simulink library "LibraryBlock"  (R2017b)
settings: Solver=VariableStepAuto  StartTime=0.0  StopTime=10.0  RelTol=1e-3
settings Model: Creator=minh  LastModifiedBy=minh

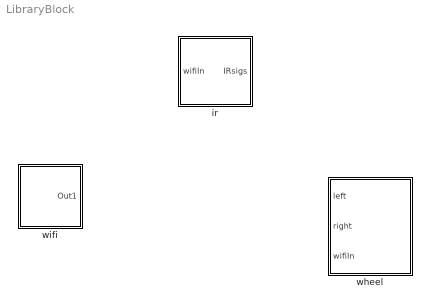
== system LibraryBlock ==
  "ir " : Subsystem
  wheel : Subsystem
  wifi : Subsystem

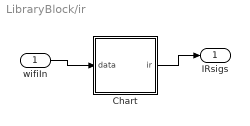
== system LibraryBlock/ir  ==
  wifiIn : Inport
  Chart : Stateflow chart  TreatAsAtomicUnit=on
  IRsigs : Outport
  wires:
  wifiIn/1 -> Chart/1(data)
  Chart/1(ir) -> IRsigs/1

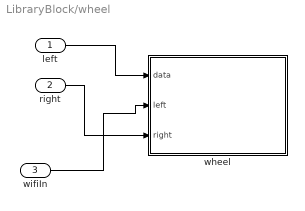
== system LibraryBlock/wheel ==
  left : Inport
  right : Inport  Port=2
  wifiIn : Inport  Port=3
  wheel : Stateflow chart  TreatAsAtomicUnit=on
  wires:
  left/1 -> wheel/1(data)
  right/1 -> wheel/3(right)
  wifiIn/1 -> wheel/2(left)

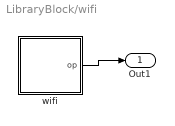
== system LibraryBlock/wifi ==
  wifi : Stateflow chart  TreatAsAtomicUnit=on
  Out1 : Outport
  wires:
  wifi/1(op) -> Out1/1

== stateflow chart LibraryBlock/wheel/wheel ==
  state f
    entry,during:
    wheel(right,left)
  (default) -> f
  data: u1 function_input; u2 function_input; data input; left input; right input
  function wheel(u1,u2):
    | function wheel(u1,u2)
    | persistent df
    | coder.extrinsic('evalin');
    | if isempty(df)
    |     df=evalin('base','re')
    | end
    | coder.extrinsic('SetWheelVelRoomba')
    | SetWheelVelRoomba(df,u1,u2)

== stateflow chart LibraryBlock/wifi/wifi ==
  state b
    entry,during:
    tcpint;
    op=0;
  (default) -> b
  data: op output
  function tcpint:
    | function tcpint
    | persistent obj
    | coder.extrinsic('RoomBaWiFi')
    | coder.extrinsic('assignin');
    | if isempty(obj)
    |     obj=RoomBaWiFi('10.0.0.1','full')
    | end
    | assignin('base','re',obj)

== stateflow chart LibraryBlock/ir /Chart ==
  state tf
    en,du:
    ir=IR;
  (default) -> tf
  data: y function_output; ir output; data input
  function y=IR:
    | function y=IR
    | y=[0,0,0,0,0,0,];
    | persistent obj
    | coder.extrinsic('evalin');
    | coder.extrinsic('get');
    | if isempty(obj)
    |     obj=evalin('base','re');
    | end
    | coder.extrinsic('RangeStateRoomba');
    | y=RangeStateRoomba(obj);
